simulink model "untitled"  (R2020b)
settings: Solver=VariableStepAuto  StartTime=0.0  StopTime=10.0  RelTol=1e-3
libraries: cstblocks x2
settings Model: Creator=salvo  LastModifiedBy=salvo

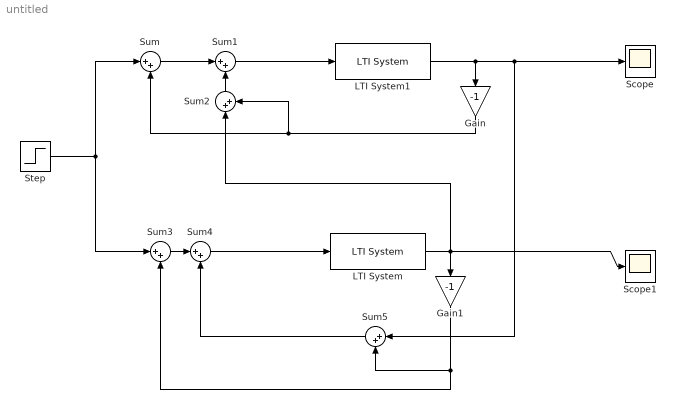
== system untitled ==
  Gain : Gain  Gain=-1
  Gain1 : Gain  Gain=-1
  LTI System : cstblocks/LTI System  sys=G  IC=[]
  LTI System1 : cstblocks/LTI System  sys=G  IC=[]
  Scope : Scope
  Scope1 : Scope
  Step : Step  SampleTime=0
  Sum{,1..5} (6 alike) : Sum  Inputs=|++
  wires:
  LTI System1/1 -> Sum5/1, Scope/1, Gain/1
  Gain/1 -> Sum/2, Sum2/2
  Sum/1 -> Sum1/1
  LTI System/1 -> Sum2/1, Gain1/1, Scope1/1
  Sum2/1 -> Sum1/2
  Sum1/1 -> LTI System1/1
  Step/1 -> Sum3/1, Sum/1
  Sum4/1 -> LTI System/1
  Gain1/1 -> Sum3/2, Sum5/2
  Sum5/1 -> Sum4/2
  Sum3/1 -> Sum4/1
